simulink model "debug_ExternalForces"  (Simulink 9.0)
settings: Solver=FixedStepDiscrete  StartTime=0.0  StopTime=inf  FixedStep=0.01  RelTol=1e-3  EnableMultiTasking=on
InitFcn:
  | ROBOT_DOF=23;
libraries: WBToolboxLibrary x7
settings Model: SuppressorTable=22 serialization::archive 11 0 6 0 0 0 11 0  Creator=DanielePucci  LastModifiedBy=icub
settings DataIOCC: LimitDataPoints=on  SaveFormat=Dataset
settings DebuggingCC: UnderspecifiedInitializationDetection=Simplified  MergeDetectMultiDrivingBlocksExec=error  AllowSymbolicDim=off
settings HardwareCC: ProdBitPerPointer=64  ProdBitPerSizeT=64  ProdBitPerPtrDiffT=64  ProdLargestAtomicFloat=Float  ProdIntDivRoundTo=Zero  ProdEndianess=LittleEndian  ProdWordSize=64  ProdHWDeviceType=Intel->x86-64 (Windows64)

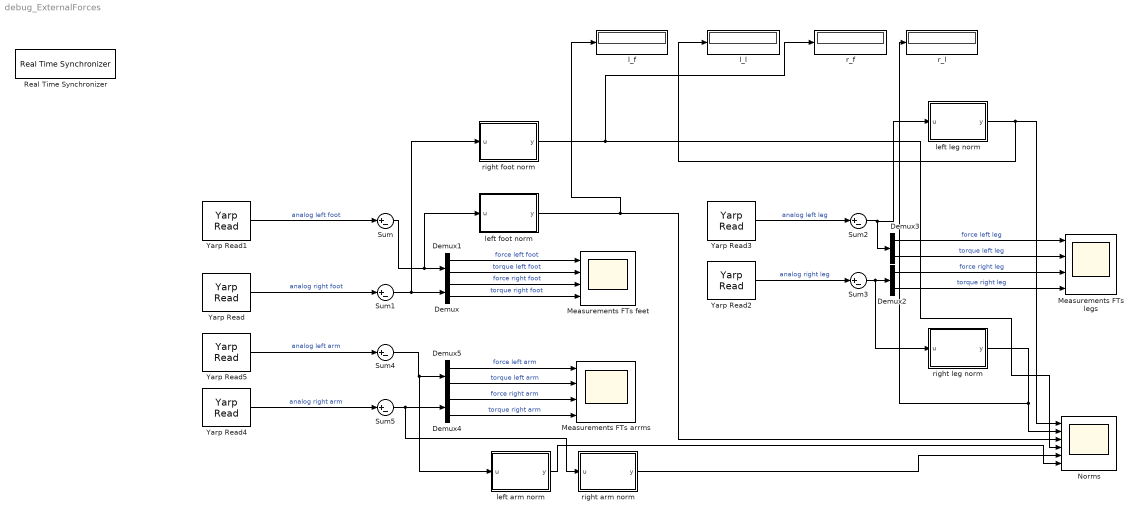
== system debug_ExternalForces ==
  Demux{,1..5} (6 alike) : Demux  Outputs=2
  Measurements FTs arrms : Scope  NumInputPorts=4
  Measurements FTs feet : Scope  NumInputPorts=4
  Measurements FTs legs : Scope  NumInputPorts=4
  Norms : Scope  NumInputPorts=6
  Real Time Synchronizer : WBToolboxLibrary/Utilities/Real Time Synchronizer  period=0.01
      settings: SourceProductName=Whole Body Toolbox
  Sum{,1..5} (6 alike) : Sum  Inputs=|+-
  Yarp Read : WBToolboxLibrary/Utilities/Yarp Read  portName='/wholeBodyDynamics/right_foot/cartesianEndEffectorWrench:o'  signalSize=6  timeout=0.5  blocking=off  timestamp=off  autoconnect=on  errorOnConnection=off
      settings: SourceProductName=Whole Body Toolbox
  Yarp Read1 : WBToolboxLibrary/Utilities/Yarp Read  portName='/wholeBodyDynamics/left_foot/cartesianEndEffectorWrench:o'  signalSize=6  timeout=0.5  blocking=off  timestamp=off  autoconnect=on  errorOnConnection=off
      settings: SourceProductName=Whole Body Toolbox
  Yarp Read2 : WBToolboxLibrary/Utilities/Yarp Read  portName='/wholeBodyDynamics/right_leg/cartesianEndEffectorWrench:o'  signalSize=6  timeout=0.5  blocking=off  timestamp=off  autoconnect=on  errorOnConnection=off
      settings: SourceProductName=Whole Body Toolbox
  Yarp Read3 : WBToolboxLibrary/Utilities/Yarp Read  portName='/wholeBodyDynamics/left_leg/cartesianEndEffectorWrench:o'  signalSize=6  timeout=0.5  blocking=off  timestamp=off  autoconnect=on  errorOnConnection=off
      settings: SourceProductName=Whole Body Toolbox
  Yarp Read4 : WBToolboxLibrary/Utilities/Yarp Read  portName='/wholeBodyDynamics/right_arm/cartesianEndEffectorWrench:o'  signalSize=6  timeout=0.5  blocking=off  timestamp=off  autoconnect=on  errorOnConnection=off
      settings: SourceProductName=Whole Body Toolbox
  Yarp Read5 : WBToolboxLibrary/Utilities/Yarp Read  portName='/wholeBodyDynamics/left_arm/cartesianEndEffectorWrench:o'  signalSize=6  timeout=0.5  blocking=off  timestamp=off  autoconnect=on  errorOnConnection=off
      settings: SourceProductName=Whole Body Toolbox
  l_f : Display
  l_l : Display
  left arm norm : MATLAB Function  TreatAsAtomicUnit=on
  left foot norm : MATLAB Function  TreatAsAtomicUnit=on
  left leg norm : MATLAB Function  TreatAsAtomicUnit=on
  r_f : Display
  r_l : Display
  "right arm norm " : MATLAB Function  TreatAsAtomicUnit=on
  "right foot norm " : MATLAB Function  TreatAsAtomicUnit=on
  right leg norm : MATLAB Function  TreatAsAtomicUnit=on
  wires:
  Yarp Read/1 -> Sum1/1  "analog right foot"
  Demux/1 -> Measurements FTs feet/3  "force right foot"
  Demux/2 -> Measurements FTs feet/4  "torque right foot"
  Yarp Read1/1 -> Sum/1  "analog left foot"
  Demux1/1 -> Measurements FTs feet/1  "force left foot"
  Demux1/2 -> Measurements FTs feet/2  "torque left foot"
  Sum/1 -> left foot norm/1(u), Demux1/1
  Sum1/1 -> "right foot norm "/1(u), Demux/1
  Yarp Read2/1 -> Sum3/1  "analog right leg"
  Demux2/1 -> Measurements FTs legs/3  "force right leg"
  Demux2/2 -> Measurements FTs legs/4  "torque right leg"
  Yarp Read3/1 -> Sum2/1  "analog left leg"
  Demux3/1 -> Measurements FTs legs/1  "force left leg"
  Demux3/2 -> Measurements FTs legs/2  "torque left leg"
  Sum2/1 -> left leg norm/1(u), Demux3/1
  Sum3/1 -> right leg norm/1(u), Demux2/1
  Yarp Read4/1 -> Sum5/1  "analog right arm"
  Demux4/1 -> Measurements FTs arrms/3  "force right arm"
  Demux4/2 -> Measurements FTs arrms/4  "torque right arm"
  Yarp Read5/1 -> Sum4/1  "analog left arm"
  Demux5/1 -> Measurements FTs arrms/1  "force left arm"
  Demux5/2 -> Measurements FTs arrms/2  "torque left arm"
  Sum4/1 -> left arm norm/1(u), Demux5/1
  Sum5/1 -> "right arm norm "/1(u), Demux4/1
  "right arm norm "/1(y) -> Norms/5
  left arm norm/1(y) -> Norms/6
  "right foot norm "/1(y) -> r_f/1, Norms/4
  left foot norm/1(y) -> l_f/1, Norms/3
  right leg norm/1(y) -> r_l/1, Norms/2
  left leg norm/1(y) -> l_l/1, Norms/1

== matlab function right arm norm  ==
  data: u input double; y output double
function y = fcn(u)
y=norm(u);

== matlab function right foot norm  ==
  data: u input double; y output double
function y = fcn(u)
y=norm(u);

== matlab function left leg norm ==
  data: u input double; y output double
function y = fcn(u)
y=norm(u);

== matlab function left arm norm ==
  data: u input double; y output double
function y = fcn(u)
y=norm(u);

== matlab function right leg norm ==
  data: u input double; y output double
function y = fcn(u)
y=norm(u);

== matlab function left foot norm ==
  data: u input double; y output double
function y = fcn(u)
y=norm(u);
